simulink model "YMC_vicrt"  (R2021a)
settings: Solver=ode4  StartTime=0.0  StopTime=inf  FixedStep=0.001  RelTol=1e-3
model workspace (MAT data in the model file):
  inChnlList : object (value not decoded)
  inChnlListInternal : object (value not decoded)
  outChnlList : object (value not decoded)
  outChnlListInternal : object (value not decoded)
values from neighbouring files (symbols this model uses):
  a = (1-wb)*w    (= 0.84425)    [YMC_launcherVICRT.m]
  b = w-a    (= 0.69075)    [YMC_launcherVICRT.m]
  BP = 1*2*pi    (= 6.28318530718)    [YMC_launcherVICRT.m]
  brakeVector = throttleVector    [YMC_launcherVICRT.m]    (also in motorMaps.m)
  Cf = 515.7027*180/pi    (= 29547.5881935)    [YMC_launcherVICRT.m]
  Cr = 630.3033*180/pi    (= 36113.7189032)    [YMC_launcherVICRT.m]
  g = 9.81    [YMC_launcherVICRT.m]
  Izz = 112.4    [YMC_launcherVICRT.m]
  m = 272    [YMC_launcherVICRT.m]
  maxYMC = maxForceAtWheel *0.4 * (tFront + tRear)    (= 1272.43505906)    [YMC_launcherVICRT.m]
  nominalWheelRadius = 0.2032    [YMC_launcherVICRT.m]
  omegaLP = 2*pi*freqLP    (= 157.079632679)    [YMC_launcherVICRT.m]
  phaseMargin = deg2rad(90)    [YMC_launcherVICRT.m]
  speedVector = linspace(0,wmax,nPoints)    [YMC_launcherVICRT.m]    (also in motorMaps.m = linspace(0,mot.limit.wmax,nPoints))
  steerFront = [-95 -92.2857142857 -89.5714285714 -86.8571428571 -84.1428571429 -81.4285714286 -78.7142857143 -76 -73.2857142857 -70.5714285714 -67.8571428571 -65.1428571429 ... (213 elements, 71x3)]    [steerFront.mat]
  taregtKUS = 0.02    [YMC_launcherVICRT.m]
  tau = 12.667    [YMC_launcherVICRT.m]
  Tc = 1e-3    (= 0.001)    [YMC_launcherVICRT.m]
  tFront = 1.23    [YMC_launcherVICRT.m]
  TorqueFront = TorqueRear * vehicle.setup.frontTorqueFactor    [motorMaps.m]    (also in torqueMaps.mat = [0 0 0 0 0 0 0 0 0 0 0 0 ... (1071 elements, 51x21)])
  TorqueFrontRegen = zeros(nPoints,nPointsPedals)    [motorMaps.m]    (also in torqueMaps.mat = [0 0 0 0 0 0 0 0 0 0 0 0 ... (1071 elements, 51x21)])
  TorqueLimit = zeros(nPoints,1)    [motorMaps.m]    (also in torqueMaps.mat = [21 21 21 21 21 21 21 21 21 21 21 21 ... (51 elements, 51x1))
  TorqueRear = zeros(nPoints,nPointsPedals)    [motorMaps.m]    (also in torqueMaps.mat = [0 0 0 0 0 0 0 0 0 0 0 0 ... (1071 elements, 51x21)])
  TorqueRearRegen = TorqueFrontRegen * vehicle.setup.rearRegenFactor    [motorMaps.m]    (also in torqueMaps.mat = [0 0 0 0 0 0 0 0 0 0 0 0 ... (1071 elements, 51x21)])
  tRear = 1.2    [YMC_launcherVICRT.m]
  w = 1.535    [YMC_launcherVICRT.m]
undefined symbols (not defined in the file or in its folder): ki, kp
libraries: simwbSfunlib x42, slpidlib x1
settings Model: Creator=Alber  LastModifiedBy=User
settings DataIOCC: ReturnWorkspaceOutputsName=outVICRT
settings DebuggingCC: UnconnectedInputMsg=none  UnconnectedOutputMsg=none  UnconnectedLineMsg=none
settings ModelReferenceCC: EnableRefExpFcnMdlSchedulingChecks=off
settings RTWCC: Description=VI-CarRealTime Solver Plugin V1.0  SystemTargetFile=vicrt_plugin.tlc  TemplateMakefile=vicrt_plugin_mingw64.tmf  PostCodeGenCommand=if strcmp(get_param(bdroot,'TemplateMakefile'),'vicrt_plugin_ccur.tmf'),copyfile([matlabroot,filesep,'rtw',filesep,'c',filesep,'tools',filesep,'unixtools.mk'],'unixtools.mk'),if ~verLessThan('matlab','9.6'),set_param(bdroot,'MatFileLogging','off'),end,end  DLArmComputeVersion=20.02.1
settings CodeAppCC: MaxIdLength=80
settings STFCustomTargetCC: TargetLangStandard=C99 (ISO)  ModelReferenceCompliant=off  CombineOutputUpdateFcns=on  MatFileLogging=on  GRTInterface=off  UseToolchainInfoCompliant=off  SystemTargetFile=vicrt_plugin.tlc
settings GRTTargetCC: ModelReferenceCompliant=off  ParMdlRefBuildCompliant=off  CompOptLevelCompliant=off  ConcurrentExecutionCompliant=off  CPPClassGenCompliant=off  UseToolchainInfoCompliant=off  RTWCAPIParams=on

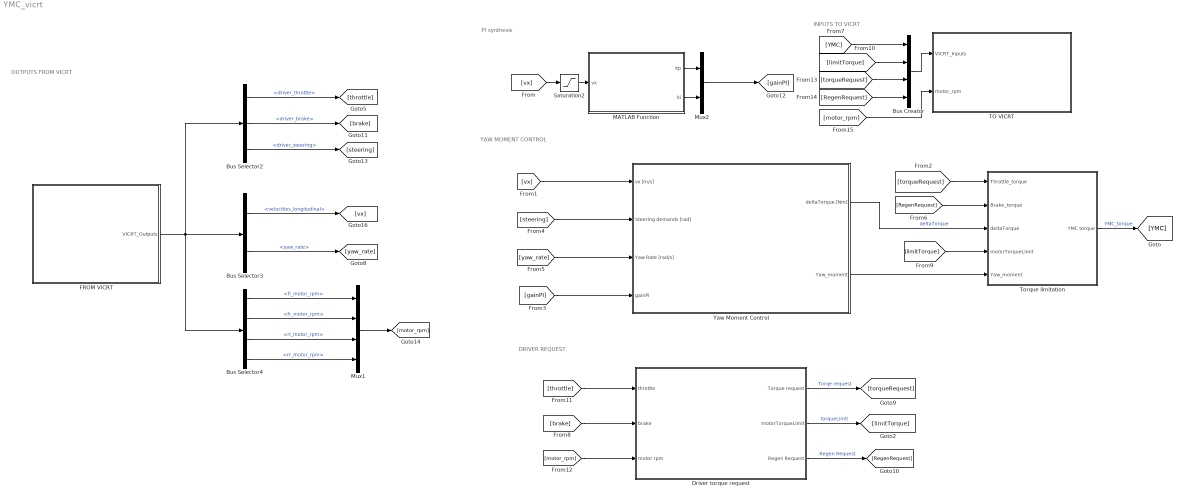
== system YMC_vicrt ==
  note: INPUTS TO VICRT
  note: OUTPUTS FROM VICRT
  note: PI synthesis
  note: DRIVER REQUEST
  note: YAW MOMENT CONTROL
  Bus Creator : BusCreator  Inputs=4
  Bus Selector2 : BusSelector  OutputSignals=driver_throttle,driver_brake,driver_steering
  Bus Selector3 : BusSelector  OutputSignals=velocities_longitudinal,yaw_rate
  Bus Selector4 : BusSelector  OutputSignals=fl_motor_rpm,fr_motor_rpm,rl_motor_rpm,rr_motor_rpm
  Driver torque request : Subsystem
  FROM VICRT : Subsystem
  MATLAB Function : MATLAB Function  TreatAsAtomicUnit=on
  Mux1 : Mux
  Mux2 : Mux  Inputs=2
  Saturation2 : Saturate  UpperLimit=inf  LowerLimit=1
  TO VICRT : Subsystem
  Torque limitation : Subsystem
  Yaw Moment Control : Subsystem
  wires:
  Driver torque request/2(motorTorqueLimit) -> [limitTorque]  "torqueLimit"
  MATLAB Function/2(ki) -> Mux2/2
  MATLAB Function/1(kp) -> Mux2/1
  Yaw Moment Control/1(deltaTorque [Nm]) -> Torque limitation/3(deltaTorque)  "deltaTorque"
  Torque limitation/1(YMC torque) -> [YMC]  "YMC_torque"
  [limitTorque] -> Torque limitation/4(motorTorqueLimit)
  Driver torque request/1(Torque request) -> [torqueRequest]  "Torqe request"
  Mux2/1 -> [gainPI]
  [vx] -> Saturation2/1
  Saturation2/1 -> MATLAB Function/1(vx)
  [gainPI] -> Yaw Moment Control/4("gainPI ")
  Bus Selector2/1 -> [throttle]  "<driver_throttle>"
  Bus Selector2/2 -> [brake]  "<driver_brake>"
  Bus Selector2/3 -> [steering]  "<driver_steering>"
  Bus Selector3/1 -> [vx]  "<velocities_longitudinal>"
  Bus Selector3/2 -> [yaw_rate]  "<yaw_rate>"
  FROM VICRT/1(VICRT_Outputs) -> Bus Selector4/1, Bus Selector3/1, Bus Selector2/1
  Bus Selector4/3 -> Mux1/3  "<rl_motor_rpm>"
  Bus Selector4/1 -> Mux1/1  "<fl_motor_rpm>"
  Bus Selector4/2 -> Mux1/2  "<fr_motor_rpm>"
  Bus Selector4/4 -> Mux1/4  "<rr_motor_rpm>"
  Mux1/1 -> [motor_rpm]
  [vx] -> Yaw Moment Control/1(vx [m/s])
  [yaw_rate] -> Yaw Moment Control/3(Yaw Rate [rad/s])
  [steering] -> Yaw Moment Control/2(Steering demands [rad])
  Driver torque request/3(Regen Request) -> [RegenRequest]  "Regen Request"
  [brake] -> Driver torque request/2(brake)
  [throttle] -> Driver torque request/1(throttle)
  [motor_rpm] -> Driver torque request/3(motor rpm)
  [torqueRequest] -> Torque limitation/1(Throttle_torque)
  [RegenRequest] -> Torque limitation/2(Brake_torque)
  [YMC] -> Bus Creator/1
  Bus Creator/1 -> TO VICRT/1(VICRT_Inputs)
  [limitTorque] -> Bus Creator/2
  Yaw Moment Control/2(Yaw_moment) -> Torque limitation/5(Yaw_moment)
  [torqueRequest] -> Bus Creator/3
  [RegenRequest] -> Bus Creator/4
  [motor_rpm] -> TO VICRT/2(motor_rpm)

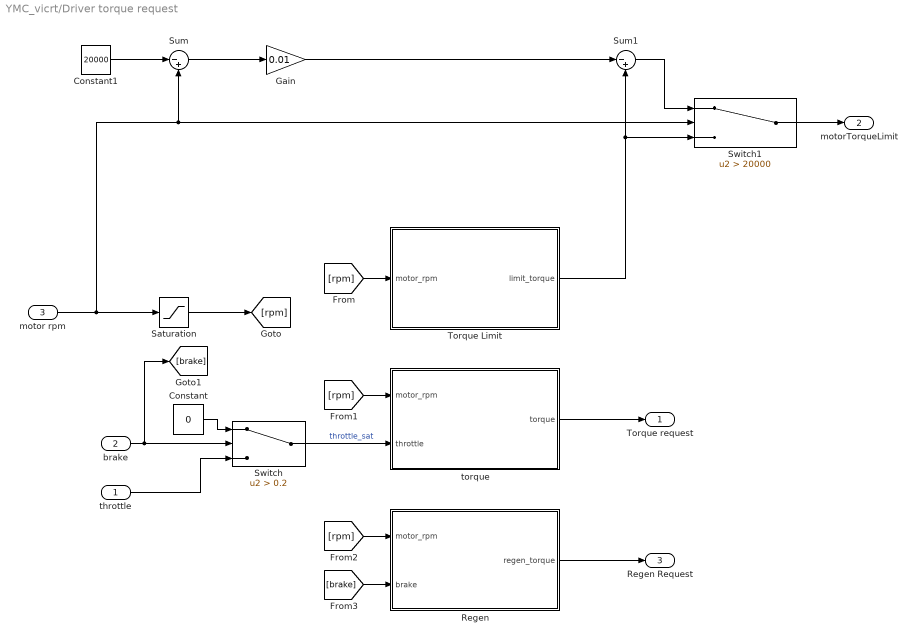
== system YMC_vicrt/Driver torque request ==
  throttle : Inport
  brake : Inport  Port=2
  motor rpm : Inport  Port=3
  Constant : Constant  Value=0
  Constant1 : Constant  Value=20000
  Gain : Gain  Gain=0.01
  Regen : Subsystem
  Saturation : Saturate  UpperLimit=20000  LowerLimit=0
  Sum : Sum  Inputs=|-+
  Sum1 : Sum  Inputs=|-+
  Switch : Switch  Criteria=u2 > Threshold  Threshold=0.2
  Switch1 : Switch  Criteria=u2 > Threshold  Threshold=20000
  Torque Limit : Subsystem
  torque : Subsystem
  Torque request : Outport
  motorTorqueLimit : Outport  Port=2
  Regen Request : Outport  Port=3
  wires:
  motor rpm/1 -> Sum/2, Switch1/2, Saturation/1
  [rpm] -> Torque Limit/1(motor_rpm)
  [rpm] -> torque/1(motor_rpm)
  [rpm] -> Regen/1(motor_rpm)
  Regen/1(regen_torque) -> Regen Request/1
  torque/1(torque) -> Torque request/1
  brake/1 -> Switch/2, [brake]
  Switch/1 -> torque/2(throttle)  "throttle_sat"
  [brake] -> Regen/2(brake)
  throttle/1 -> Switch/3
  Constant/1 -> Switch/1
  Saturation/1 -> [rpm]
  Constant1/1 -> Sum/1
  Sum/1 -> Gain/1
  Gain/1 -> Sum1/1
  Sum1/1 -> Switch1/1
  Switch1/1 -> motorTorqueLimit/1
  Torque Limit/1(limit_torque) -> Switch1/3, Sum1/2

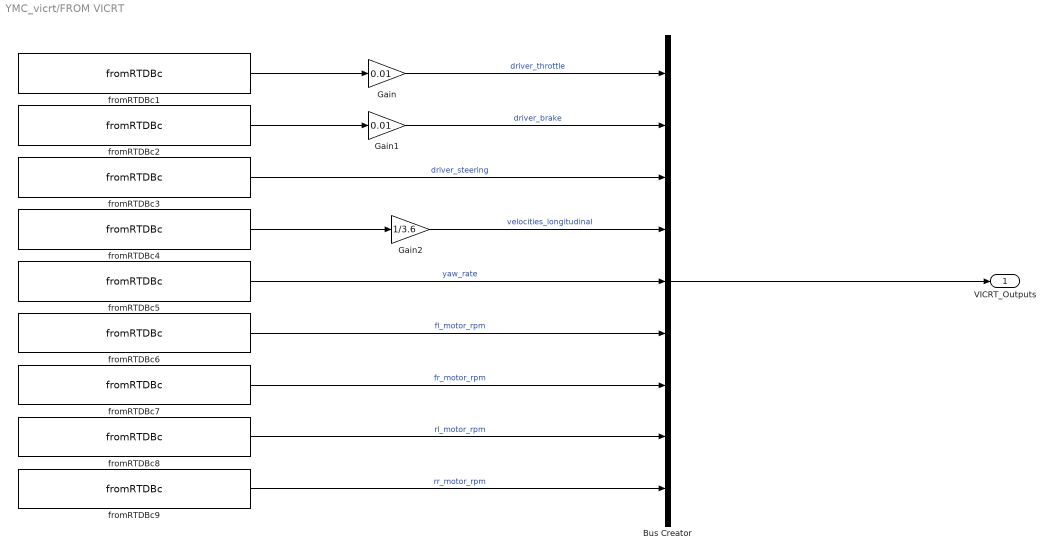
== system YMC_vicrt/FROM VICRT ==
  Bus Creator : BusCreator  Inputs=9
  Gain : Gain  Gain=0.01
  Gain1 : Gain  Gain=0.01
  Gain2 : Gain  Gain=1/3.6
  fromRTDBc1 : simwbSfunlib/fromRTDBc  stringBlock=off  varName=VI_CarRealTime.Outputs.driver_demands.throttle  sigDim=[1 1]  sigType=double  sampleTime=[-1 0]  maxBuffSize=1024  busName=nobus  defaultValue=0  defaultString=simwbin  hasMapping=0  ptrName=VI_CarRealTime_Outputs_driver_demands_throttle  enumOrAlias=nothing
      settings: SourceProductName=SimWB MLToolkit
  fromRTDBc2 : simwbSfunlib/fromRTDBc  stringBlock=off  varName=VI_CarRealTime.Outputs.driver_demands.brake  sigDim=[1 1]  sigType=double  sampleTime=[-1 0]  maxBuffSize=1024  busName=nobus  defaultValue=0  defaultString=simwbin  hasMapping=0  ptrName=VI_CarRealTime_Outputs_driver_demands_brake  enumOrAlias=nothing
      settings: SourceProductName=SimWB MLToolkit
  fromRTDBc3 : simwbSfunlib/fromRTDBc  stringBlock=off  varName=VI_CarRealTime.Outputs.driver_demands.steering  sigDim=[1 1]  sigType=double  sampleTime=[-1 0]  maxBuffSize=1024  busName=nobus  defaultValue=0  defaultString=simwbin  hasMapping=0  ptrName=VI_CarRealTime_Outputs_driver_demands_steering  enumOrAlias=nothing
      settings: SourceProductName=SimWB MLToolkit
  fromRTDBc4 : simwbSfunlib/fromRTDBc  stringBlock=off  varName=VI_CarRealTime.Outputs.chassis_velocities.longitudinal  sigDim=[1 1]  sigType=double  sampleTime=[-1 0]  maxBuffSize=1024  busName=nobus  defaultValue=0  defaultString=simwbin  hasMapping=0  ptrName=VI_CarRealTime_Outputs_chassis_velocities_longitudinal  enumOrAlias=nothing
      settings: SourceProductName=SimWB MLToolkit
  fromRTDBc5 : simwbSfunlib/fromRTDBc  stringBlock=off  varName=VI_CarRealTime.Outputs.chassis_velocities.yaw  sigDim=[1 1]  sigType=double  sampleTime=[-1 0]  maxBuffSize=1024  busName=nobus  defaultValue=0  defaultString=simwbin  hasMapping=0  ptrName=VI_CarRealTime_Outputs_chassis_velocities_yaw  enumOrAlias=nothing
      settings: SourceProductName=SimWB MLToolkit
  fromRTDBc6 : simwbSfunlib/fromRTDBc  stringBlock=off  varName=VI_CarRealTime.Outputs.motor_to_front_left_wheel.engine_rpm  sigDim=[1 1]  sigType=double  sampleTime=[-1 0]  maxBuffSize=1024  busName=nobus  defaultValue=0  defaultString=simwbin  hasMapping=0  ptrName=VI_CarRealTime_Outputs_motor_to_front_left_wheel_engine_rpm  enumOrAlias=nothing
      settings: SourceProductName=SimWB MLToolkit
  fromRTDBc7 : simwbSfunlib/fromRTDBc  stringBlock=off  varName=VI_CarRealTime.Outputs.motor_to_front_right_wheel.engine_rpm  sigDim=[1 1]  sigType=double  sampleTime=[-1 0]  maxBuffSize=1024  busName=nobus  defaultValue=0  defaultString=simwbin  hasMapping=0  ptrName=VI_CarRealTime_Outputs_motor_to_front_right_wheel_engine_rpm  enumOrAlias=nothing
      settings: SourceProductName=SimWB MLToolkit
  fromRTDBc8 : simwbSfunlib/fromRTDBc  stringBlock=off  varName=VI_CarRealTime.Outputs.motor_to_rear_left_wheel.engine_rpm  sigDim=[1 1]  sigType=double  sampleTime=[-1 0]  maxBuffSize=1024  busName=nobus  defaultValue=0  defaultString=simwbin  hasMapping=0  ptrName=VI_CarRealTime_Outputs_motor_to_rear_left_wheel_engine_rpm  enumOrAlias=nothing
      settings: SourceProductName=SimWB MLToolkit
  fromRTDBc9 : simwbSfunlib/fromRTDBc  stringBlock=off  varName=VI_CarRealTime.Outputs.motor_to_rear_right_wheel.engine_rpm  sigDim=[1 1]  sigType=double  sampleTime=[-1 0]  maxBuffSize=1024  busName=nobus  defaultValue=0  defaultString=simwbin  hasMapping=0  ptrName=VI_CarRealTime_Outputs_motor_to_rear_right_wheel_engine_rpm  enumOrAlias=nothing
      settings: SourceProductName=SimWB MLToolkit
  VICRT_Outputs : Outport
  wires:
  Bus Creator/1 -> VICRT_Outputs/1
  fromRTDBc1/1 -> Gain/1
  Gain/1 -> Bus Creator/1  "driver_throttle"
  fromRTDBc2/1 -> Gain1/1
  Gain1/1 -> Bus Creator/2  "driver_brake"
  fromRTDBc3/1 -> Bus Creator/3  "driver_steering"
  fromRTDBc5/1 -> Bus Creator/5  "yaw_rate"
  fromRTDBc4/1 -> Gain2/1
  Gain2/1 -> Bus Creator/4  "velocities_longitudinal"
  fromRTDBc6/1 -> Bus Creator/6  "fl_motor_rpm"
  fromRTDBc7/1 -> Bus Creator/7  "fr_motor_rpm"
  fromRTDBc8/1 -> Bus Creator/8  "rl_motor_rpm"
  fromRTDBc9/1 -> Bus Creator/9  "rr_motor_rpm"

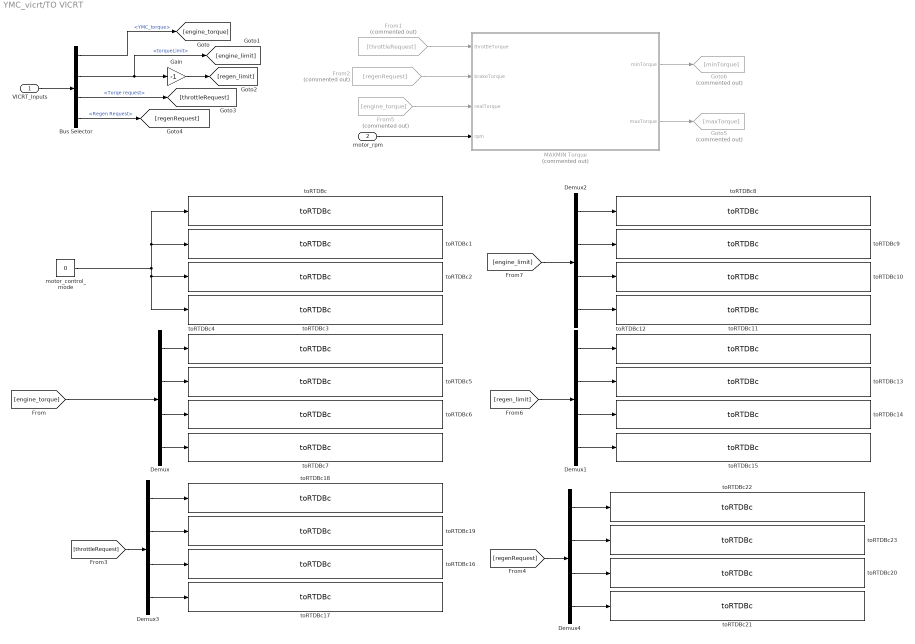
== system YMC_vicrt/TO VICRT ==
  VICRT_Inputs : Inport
  motor_rpm : Inport  Port=2
  Bus Selector : BusSelector  OutputSignals=YMC_torque,torqueLimit,Torqe request,Regen Request
  Demux{,1..4} (5 alike) : Demux
  From1 : From  Commented=on  GotoTag=throttleRequest
  From2 : From  Commented=on  GotoTag=regenRequest
  From5 : From  Commented=on  GotoTag=engine_torque
  Gain : Gain  Gain=-1
  Goto5 : Goto  Commented=on  GotoTag=maxTorque
  Goto6 : Goto  Commented=on  GotoTag=minTorque
  MAXMIN Torque : Subsystem  Commented=on
  motor_control_mode : Constant  Value=0
  toRTDBc : simwbSfunlib/toRTDBc  stringBlock=off  varName=VI_CarRealTime.Inputs.Subsystem_Activation.Internal_Motor_to_FrontLeftWheel_Activity  sigDim=[1 1]  sigType=double  sampleTime=[-1 0]  maxBuffSize=1024  busName=nobus  defaultValue=0  defaultString=simwbout  hasMapping=0  ptrName=VI_CarRealTime_Inputs_Subsystem_Activation_Internal_Motor_to_FrontLeftWheel_Activity  enumOrAlias=nothing
      settings: SourceProductName=SimWB MLToolkit
  toRTDBc1 : simwbSfunlib/toRTDBc  stringBlock=off  varName=VI_CarRealTime.Inputs.Subsystem_Activation.Internal_Motor_to_FrontRightWheel_Activity  sigDim=[1 1]  sigType=double  sampleTime=[-1 0]  maxBuffSize=1024  busName=nobus  defaultValue=0  defaultString=simwbout  hasMapping=0  ptrName=VI_CarRealTime_Inputs_Subsystem_Activation_Internal_Motor_to_FrontRightWheel_Activity  enumOrAlias=nothing
      settings: SourceProductName=SimWB MLToolkit
  toRTDBc10 : simwbSfunlib/toRTDBc  stringBlock=off  varName=VI_CarRealTime.Inputs.Generic_Engine_to_Rear_Left_Wheel.engine_max_torque  sigDim=[1 1]  sigType=double  sampleTime=[-1 0]  maxBuffSize=1024  busName=nobus  defaultValue=0  defaultString=simwbout  hasMapping=0  ptrName=VI_CarRealTime_Inputs_Generic_Engine_to_Rear_Left_Wheel_engine_max_torque  enumOrAlias=nothing
      settings: SourceProductName=SimWB MLToolkit
  toRTDBc11 : simwbSfunlib/toRTDBc  stringBlock=off  varName=VI_CarRealTime.Inputs.Generic_Engine_to_Rear_Right_Wheel.engine_max_torque  sigDim=[1 1]  sigType=double  sampleTime=[-1 0]  maxBuffSize=1024  busName=nobus  defaultValue=0  defaultString=simwbout  hasMapping=0  ptrName=VI_CarRealTime_Inputs_Generic_Engine_to_Rear_Right_Wheel_engine_max_torque  enumOrAlias=nothing
      settings: SourceProductName=SimWB MLToolkit
  toRTDBc12 : simwbSfunlib/toRTDBc  stringBlock=off  varName=VI_CarRealTime.Inputs.Generic_Engine_to_Front_Left_Wheel.engine_min_torque  sigDim=[1 1]  sigType=double  sampleTime=[-1 0]  maxBuffSize=1024  busName=nobus  defaultValue=0  defaultString=simwbout  hasMapping=0  ptrName=VI_CarRealTime_Inputs_Generic_Engine_to_Front_Left_Wheel_engine_min_torque  enumOrAlias=nothing
      settings: SourceProductName=SimWB MLToolkit
  toRTDBc13 : simwbSfunlib/toRTDBc  stringBlock=off  varName=VI_CarRealTime.Inputs.Generic_Engine_to_Front_Right_Wheel.engine_min_torque  sigDim=[1 1]  sigType=double  sampleTime=[-1 0]  maxBuffSize=1024  busName=nobus  defaultValue=0  defaultString=simwbout  hasMapping=0  ptrName=VI_CarRealTime_Inputs_Generic_Engine_to_Front_Right_Wheel_engine_min_torque  enumOrAlias=nothing
      settings: SourceProductName=SimWB MLToolkit
  toRTDBc14 : simwbSfunlib/toRTDBc  stringBlock=off  varName=VI_CarRealTime.Inputs.Generic_Engine_to_Rear_Left_Wheel.engine_min_torque  sigDim=[1 1]  sigType=double  sampleTime=[-1 0]  maxBuffSize=1024  busName=nobus  defaultValue=0  defaultString=simwbout  hasMapping=0  ptrName=VI_CarRealTime_Inputs_Generic_Engine_to_Rear_Left_Wheel_engine_min_torque  enumOrAlias=nothing
      settings: SourceProductName=SimWB MLToolkit
  toRTDBc15 : simwbSfunlib/toRTDBc  stringBlock=off  varName=VI_CarRealTime.Inputs.Generic_Engine_to_Rear_Right_Wheel.engine_min_torque  sigDim=[1 1]  sigType=double  sampleTime=[-1 0]  maxBuffSize=1024  busName=nobus  defaultValue=0  defaultString=simwbout  hasMapping=0  ptrName=VI_CarRealTime_Inputs_Generic_Engine_to_Rear_Right_Wheel_engine_min_torque  enumOrAlias=nothing
      settings: SourceProductName=SimWB MLToolkit
  toRTDBc16 : simwbSfunlib/toRTDBc  stringBlock=off  varName=YMC.torqueRequest.RL  sigDim=[1 1]  sigType=double  sampleTime=[-1 0]  maxBuffSize=1024  busName=nobus  defaultValue=0  defaultString=simwbout  hasMapping=0  ptrName=YMC_torqueRequest_RL  enumOrAlias=nothing
      settings: SourceProductName=SimWB MLToolkit
  toRTDBc17 : simwbSfunlib/toRTDBc  stringBlock=off  varName=YMC.torqueRequest.RR  sigDim=[1 1]  sigType=double  sampleTime=[-1 0]  maxBuffSize=1024  busName=nobus  defaultValue=0  defaultString=simwbout  hasMapping=0  ptrName=YMC_torqueRequest_RR  enumOrAlias=nothing
      settings: SourceProductName=SimWB MLToolkit
  toRTDBc18 : simwbSfunlib/toRTDBc  stringBlock=off  varName=YMC.torqueRequest.FL  sigDim=[1 1]  sigType=double  sampleTime=[-1 0]  maxBuffSize=1024  busName=nobus  defaultValue=0  defaultString=simwbout  hasMapping=0  ptrName=YMC_torqueRequest_FL  enumOrAlias=nothing
      settings: SourceProductName=SimWB MLToolkit
  toRTDBc19 : simwbSfunlib/toRTDBc  stringBlock=off  varName=YMC.torqueRequest.FR  sigDim=[1 1]  sigType=double  sampleTime=[-1 0]  maxBuffSize=1024  busName=nobus  defaultValue=0  defaultString=simwbout  hasMapping=0  ptrName=YMC_torqueRequest_FR  enumOrAlias=nothing
      settings: SourceProductName=SimWB MLToolkit
  toRTDBc2 : simwbSfunlib/toRTDBc  stringBlock=off  varName=VI_CarRealTime.Inputs.Subsystem_Activation.Internal_Motor_to_RearLeftWheel_Activity  sigDim=[1 1]  sigType=double  sampleTime=[-1 0]  maxBuffSize=1024  busName=nobus  defaultValue=0  defaultString=simwbout  hasMapping=0  ptrName=VI_CarRealTime_Inputs_Subsystem_Activation_Internal_Motor_to_RearLeftWheel_Activity  enumOrAlias=nothing
      settings: SourceProductName=SimWB MLToolkit
  toRTDBc20 : simwbSfunlib/toRTDBc  stringBlock=off  varName=YMC.regenRequest.RL  sigDim=[1 1]  sigType=double  sampleTime=[-1 0]  maxBuffSize=1024  busName=nobus  defaultValue=0  defaultString=simwbout  hasMapping=0  ptrName=YMC_regenRequest_RL  enumOrAlias=nothing
      settings: SourceProductName=SimWB MLToolkit
  toRTDBc21 : simwbSfunlib/toRTDBc  stringBlock=off  varName=YMC.regenRequest.RR  sigDim=[1 1]  sigType=double  sampleTime=[-1 0]  maxBuffSize=1024  busName=nobus  defaultValue=0  defaultString=simwbout  hasMapping=0  ptrName=YMC_regenRequest_RR  enumOrAlias=nothing
      settings: SourceProductName=SimWB MLToolkit
  toRTDBc22 : simwbSfunlib/toRTDBc  stringBlock=off  varName=YMC.regenRequest.FL  sigDim=[1 1]  sigType=double  sampleTime=[-1 0]  maxBuffSize=1024  busName=nobus  defaultValue=0  defaultString=simwbout  hasMapping=0  ptrName=YMC_regenRequest_FL  enumOrAlias=nothing
      settings: SourceProductName=SimWB MLToolkit
  toRTDBc23 : simwbSfunlib/toRTDBc  stringBlock=off  varName=YMC.regenRequest.FR  sigDim=[1 1]  sigType=double  sampleTime=[-1 0]  maxBuffSize=1024  busName=nobus  defaultValue=0  defaultString=simwbout  hasMapping=0  ptrName=YMC_regenRequest_FR  enumOrAlias=nothing
      settings: SourceProductName=SimWB MLToolkit
  toRTDBc3 : simwbSfunlib/toRTDBc  stringBlock=off  varName=VI_CarRealTime.Inputs.Subsystem_Activation.Internal_Motor_to_RearRightWheel_Activity  sigDim=[1 1]  sigType=double  sampleTime=[-1 0]  maxBuffSize=1024  busName=nobus  defaultValue=0  defaultString=simwbout  hasMapping=0  ptrName=VI_CarRealTime_Inputs_Subsystem_Activation_Internal_Motor_to_RearRightWheel_Activity  enumOrAlias=nothing
      settings: SourceProductName=SimWB MLToolkit
  toRTDBc4 : simwbSfunlib/toRTDBc  stringBlock=off  varName=VI_CarRealTime.Inputs.Generic_Engine_to_Front_Left_Wheel.engine_torque  sigDim=[1 1]  sigType=double  sampleTime=[-1 0]  maxBuffSize=1024  busName=nobus  defaultValue=0  defaultString=simwbout  hasMapping=0  ptrName=VI_CarRealTime_Inputs_Generic_Engine_to_Front_Left_Wheel_engine_torque  enumOrAlias=nothing
      settings: SourceProductName=SimWB MLToolkit
  toRTDBc5 : simwbSfunlib/toRTDBc  stringBlock=off  varName=VI_CarRealTime.Inputs.Generic_Engine_to_Front_Right_Wheel.engine_torque  sigDim=[1 1]  sigType=double  sampleTime=[-1 0]  maxBuffSize=1024  busName=nobus  defaultValue=0  defaultString=simwbout  hasMapping=0  ptrName=VI_CarRealTime_Inputs_Generic_Engine_to_Front_Right_Wheel_engine_torque  enumOrAlias=nothing
      settings: SourceProductName=SimWB MLToolkit
  toRTDBc6 : simwbSfunlib/toRTDBc  stringBlock=off  varName=VI_CarRealTime.Inputs.Generic_Engine_to_Rear_Left_Wheel.engine_torque  sigDim=[1 1]  sigType=double  sampleTime=[-1 0]  maxBuffSize=1024  busName=nobus  defaultValue=0  defaultString=simwbout  hasMapping=0  ptrName=VI_CarRealTime_Inputs_Generic_Engine_to_Rear_Left_Wheel_engine_torque  enumOrAlias=nothing
      settings: SourceProductName=SimWB MLToolkit
  toRTDBc7 : simwbSfunlib/toRTDBc  stringBlock=off  varName=VI_CarRealTime.Inputs.Generic_Engine_to_Rear_Right_Wheel.engine_torque  sigDim=[1 1]  sigType=double  sampleTime=[-1 0]  maxBuffSize=1024  busName=nobus  defaultValue=0  defaultString=simwbout  hasMapping=0  ptrName=VI_CarRealTime_Inputs_Generic_Engine_to_Rear_Right_Wheel_engine_torque  enumOrAlias=nothing
      settings: SourceProductName=SimWB MLToolkit
  toRTDBc8 : simwbSfunlib/toRTDBc  stringBlock=off  varName=VI_CarRealTime.Inputs.Generic_Engine_to_Front_Left_Wheel.engine_max_torque  sigDim=[1 1]  sigType=double  sampleTime=[-1 0]  maxBuffSize=1024  busName=nobus  defaultValue=0  defaultString=simwbout  hasMapping=0  ptrName=VI_CarRealTime_Inputs_Generic_Engine_to_Front_Left_Wheel_engine_max_torque  enumOrAlias=nothing
      settings: SourceProductName=SimWB MLToolkit
  toRTDBc9 : simwbSfunlib/toRTDBc  stringBlock=off  varName=VI_CarRealTime.Inputs.Generic_Engine_to_Front_Right_Wheel.engine_max_torque  sigDim=[1 1]  sigType=double  sampleTime=[-1 0]  maxBuffSize=1024  busName=nobus  defaultValue=0  defaultString=simwbout  hasMapping=0  ptrName=VI_CarRealTime_Inputs_Generic_Engine_to_Front_Right_Wheel_engine_max_torque  enumOrAlias=nothing
      settings: SourceProductName=SimWB MLToolkit
  wires:
  VICRT_Inputs/1 -> Bus Selector/1
  motor_control_mode/1 -> toRTDBc1/1, toRTDBc/1, toRTDBc3/1, toRTDBc2/1
  Bus Selector/1 -> [engine_torque]  "<YMC_torque>"
  Bus Selector/2 -> [engine_limit], Gain/1  "<torqueLimit>"
  Demux/1 -> toRTDBc4/1
  Demux/2 -> toRTDBc5/1
  Demux/3 -> toRTDBc6/1
  Demux/4 -> toRTDBc7/1
  Demux1/4 -> toRTDBc15/1
  Demux1/2 -> toRTDBc13/1
  Demux1/3 -> toRTDBc14/1
  Demux1/1 -> toRTDBc12/1
  Demux2/4 -> toRTDBc11/1
  Demux2/3 -> toRTDBc10/1
  Demux2/2 -> toRTDBc9/1
  Demux2/1 -> toRTDBc8/1
  Gain/1 -> [regen_limit]
  [regen_limit] -> Demux1/1
  [engine_limit] -> Demux2/1
  Bus Selector/3 -> [throttleRequest]  "<Torqe request>"
  Bus Selector/4 -> [regenRequest]  "<Regen Request>"
  Demux3/2 -> toRTDBc19/1
  Demux3/4 -> toRTDBc17/1
  [throttleRequest] -> Demux3/1
  Demux3/3 -> toRTDBc16/1
  Demux3/1 -> toRTDBc18/1
  Demux4/2 -> toRTDBc23/1
  Demux4/1 -> toRTDBc22/1
  Demux4/3 -> toRTDBc20/1
  [regenRequest] -> Demux4/1
  Demux4/4 -> toRTDBc21/1
  From1/1 -> MAXMIN Torque/1(throttleTorque)
  From2/1 -> MAXMIN Torque/2(brakeTorque)
  From5/1 -> MAXMIN Torque/3(realTorque)
  motor_rpm/1 -> MAXMIN Torque/4(rpm)
  MAXMIN Torque/1(minTorque) -> Goto6/1
  MAXMIN Torque/2(maxTorque) -> Goto5/1
  [engine_torque] -> Demux/1

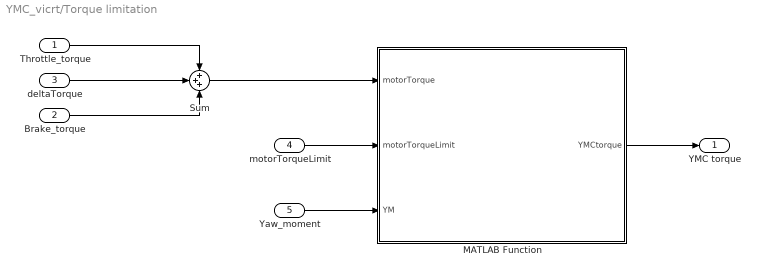
== system YMC_vicrt/Torque limitation ==
  Throttle_torque : Inport
  Brake_torque : Inport  Port=2
  deltaTorque : Inport  Port=3
  motorTorqueLimit : Inport  Port=4
  Yaw_moment : Inport  Port=5
  MATLAB Function : MATLAB Function  TreatAsAtomicUnit=on
  Sum : Sum  Inputs=+++
  YMC torque : Outport
  wires:
  motorTorqueLimit/1 -> MATLAB Function/2(motorTorqueLimit)
  Brake_torque/1 -> Sum/3
  deltaTorque/1 -> Sum/2
  Throttle_torque/1 -> Sum/1
  Sum/1 -> MATLAB Function/1(motorTorque)
  Yaw_moment/1 -> MATLAB Function/3(YM)
  MATLAB Function/1(YMCtorque) -> YMC torque/1

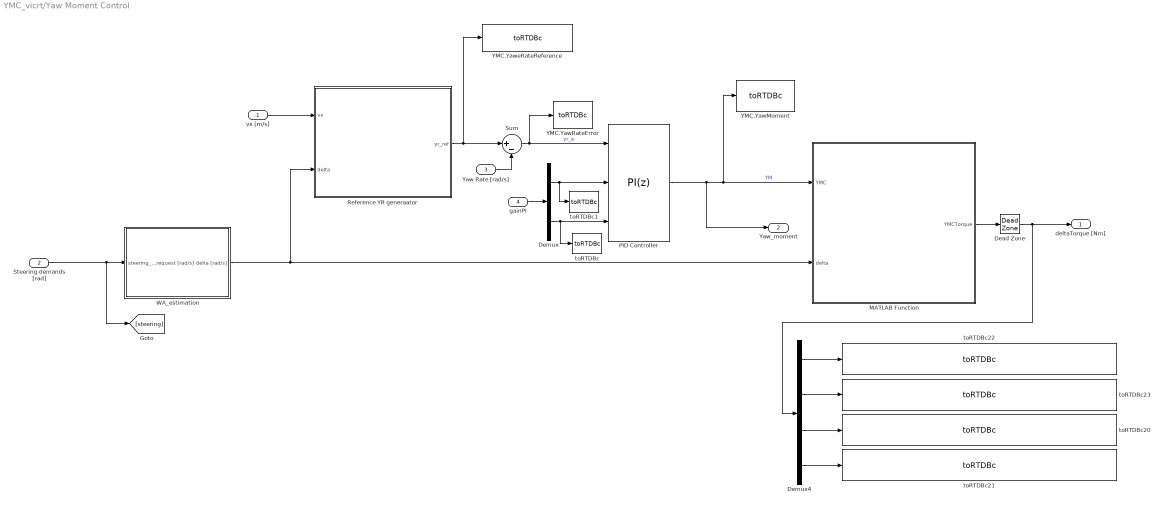
== system YMC_vicrt/Yaw Moment Control ==
  vx [m/s] : Inport
  Steering demands [rad] : Inport  Port=2
  Yaw Rate [rad/s] : Inport  Port=3
  "gainPI " : Inport  Port=4
  Dead Zone : DeadZone  LowerValue=-0.1  UpperValue=0.1  SaturateOnIntegerOverflow=on
  Demux : Demux  Outputs=2
  Demux4 : Demux
  MATLAB Function : MATLAB Function  TreatAsAtomicUnit=on
  PID Controller : slpidlib/PID Controller  Controller=PI  Form=Parallel  TimeDomain=Discrete-time  UseExternalTs=off  SampleTime=Tc  IntegratorMethod=Forward Euler  FilterMethod=Forward Euler  ControllerParametersSource=external  P=kp  I=ki  D=1  UseFilter=on  N=140.723674968444  TunerSelectOption=Transfer Function Based (PID Tuner App)  InitialConditionSource=internal  InitialConditionForIntegrator=0  InitialConditionForFilter=0  DifferentiatorICPrevScaledInput=0  ExternalReset=none  TrackingMode=off  Kt=1  LimitOutput=on  SatLimitsSource=internal  UpperSaturationLimit=1*maxYMC  LowerSaturationLimit=-1*maxYMC  LinearizeAsGain=off  AntiWindupMode=clamping  Kb=1  POutMin=[]  POutMax=[]  IOutMin=[]  IOutMax=[]  DOutMin=[]  DOutMax=[]  NOutMin=[]  NOutMax=[]  SumOutMin=[]  SumOutMax=[]  SaturationOutMin=[]  SaturationOutMax=[]  PParamMin=[]  PParamMax=[]  IParamMin=[]  IParamMax=[]  DParamMin=[]  DParamMax=[]  NParamMin=[]  NParamMax=[]  KbParamMin=[]  KbParamMax=[]  KtParamMin=[]  KtParamMax=[]  KbOutMin=[]  KbOutMax=[]  KtOutMin=[]  KtOutMax=[]  IntegratorOutMin=[]  IntegratorOutMax=[]  FilterOutMin=[]  FilterOutMax=[]  SumI1OutMin=[]  SumI1OutMax=[]  SumI2OutMin=[]  SumI2OutMax=[]  SumI3OutMin=[]  SumI3OutMax=[]  SumI4OutMin=[]  SumI4OutMax=[]  SumDOutMin=[]  SumDOutMax=[]  DifferentiatorOutMin=[]  DifferentiatorOutMax=[]  FilterDiffOutCoefMin=[]  FilterDiffOutCoefMax=[]  ReciprocalOutMin=[]  ReciprocalOutMax=[]  SumDenOutMin=[]  SumDenOutMax=[]  SumNumOutMin=[]  SumNumOutMax=[]  DivideOutMin=[]  DivideOutMax=[]  UdiffTsProdOutMin=[]  UdiffTsProdOutMax=[]  NTsProdOutMin=[]  NTsProdOutMax=[]  UintegralTsProdOutMin=[]  UintegralTsProdOutMax=[]  UngainTsProdOutMin=[]  UngainTsProdOutMax=[]  IntegratorContinuousStateAttributes=''  IntegratorStateMustResolveToSignalObject=off  IntegratorRTWStateStorageClass=Auto  FilterContinuousStateAttributes=''  FilterStateMustResolveToSignalObject=off  FilterRTWStateStorageClass=Auto  ParallelPVariant=ExternalParameters  IdealPVariant=Disabled  IVariant=ExternalParameters  DVariant=Disabled  IntegratorVariant=Discrete  SatVariant=Enabled  AWVariant=DiscClampingParallel  PCopyVariant=Disabled  TRVariant=Disabled  FdbkBlocksVariant=Forward  IdealPFdbkVariant=Disabled  SatFdbkVariant=Disabled  DerivativeFilterVariant=Disabled  NVariant=Disabled  NCopyVariant=Disabled_SignalSpec  FilterICVariant=Disabled  IntegratorICVariant=InternalICs  ExternalResetVariant=Disabled  TRSumVariant=Passthrough  SumFdbkVariant=Disabled  SumVariant=Sum_PI  TsampFilterVariant=InternalTs  TsampNgainVariant=Passthrough  TsampIntegralVariant=Passthrough  ExternalSaturationOutDataTypeStr=Inherit: Same as second input
  Reference YR generaator : Subsystem
  Sum : Sum  Inputs=|+-
  WA_estimation : Subsystem
  YMC.YawMoment : simwbSfunlib/toRTDBc  stringBlock=off  varName=YMC.YawMoment  sigDim=[1 1]  sigType=double  sampleTime=[-1 0]  maxBuffSize=1024  busName=nobus  defaultValue=0  defaultString=simwbout  hasMapping=0  ptrName=YMC_YawMoment  enumOrAlias=nothing
      settings: SourceProductName=SimWB MLToolkit
  YMC.YawRateError : simwbSfunlib/toRTDBc  stringBlock=off  varName=YMC.YawRateError  sigDim=[1 1]  sigType=double  sampleTime=[-1 0]  maxBuffSize=1024  busName=nobus  defaultValue=0  defaultString=simwbout  hasMapping=0  ptrName=YMC_YawRateError  enumOrAlias=nothing
      settings: SourceProductName=SimWB MLToolkit
  YMC.YaweRateReference : simwbSfunlib/toRTDBc  stringBlock=off  varName=YMC.YawRateReference  sigDim=[1 1]  sigType=double  sampleTime=[-1 0]  maxBuffSize=1024  busName=nobus  defaultValue=0  defaultString=simwbout  hasMapping=0  ptrName=YMC_YawRateReference  enumOrAlias=nothing
      settings: SourceProductName=SimWB MLToolkit
  toRTDBc : simwbSfunlib/toRTDBc  stringBlock=off  varName=YMC.PI.ki  sigDim=[1 1]  sigType=double  sampleTime=[-1 0]  maxBuffSize=1024  busName=nobus  defaultValue=0  defaultString=simwbout  hasMapping=0  ptrName=YMC_PI_ki  enumOrAlias=nothing
      settings: SourceProductName=SimWB MLToolkit
  toRTDBc1 : simwbSfunlib/toRTDBc  stringBlock=off  varName=YMC.PI.kp  sigDim=[1 1]  sigType=double  sampleTime=[-1 0]  maxBuffSize=1024  busName=nobus  defaultValue=0  defaultString=simwbout  hasMapping=0  ptrName=YMC_PI_kp  enumOrAlias=nothing
      settings: SourceProductName=SimWB MLToolkit
  toRTDBc20 : simwbSfunlib/toRTDBc  stringBlock=off  varName=YMC.delta.RL  sigDim=[1 1]  sigType=double  sampleTime=[-1 0]  maxBuffSize=1024  busName=nobus  defaultValue=0  defaultString=simwbout  hasMapping=0  ptrName=YMC_delta_RL  enumOrAlias=nothing
      settings: SourceProductName=SimWB MLToolkit
  toRTDBc21 : simwbSfunlib/toRTDBc  stringBlock=off  varName=YMC.delta.RR  sigDim=[1 1]  sigType=double  sampleTime=[-1 0]  maxBuffSize=1024  busName=nobus  defaultValue=0  defaultString=simwbout  hasMapping=0  ptrName=YMC_delta_RR  enumOrAlias=nothing
      settings: SourceProductName=SimWB MLToolkit
  toRTDBc22 : simwbSfunlib/toRTDBc  stringBlock=off  varName=YMC.delta.FL  sigDim=[1 1]  sigType=double  sampleTime=[-1 0]  maxBuffSize=1024  busName=nobus  defaultValue=0  defaultString=simwbout  hasMapping=0  ptrName=YMC_delta_FL  enumOrAlias=nothing
      settings: SourceProductName=SimWB MLToolkit
  toRTDBc23 : simwbSfunlib/toRTDBc  stringBlock=off  varName=YMC.delta.FR  sigDim=[1 1]  sigType=double  sampleTime=[-1 0]  maxBuffSize=1024  busName=nobus  defaultValue=0  defaultString=simwbout  hasMapping=0  ptrName=YMC_delta_FR  enumOrAlias=nothing
      settings: SourceProductName=SimWB MLToolkit
  deltaTorque [Nm] : Outport
  Yaw_moment : Outport  Port=2
  wires:
  MATLAB Function/1(YMCTorque) -> Dead Zone/1
  PID Controller/1 -> YMC.YawMoment/1, MATLAB Function/1(YMC), Yaw_moment/1  "YM"
  vx [m/s]/1 -> Reference YR generaator/1(vx)
  Reference YR generaator/1(yr_ref) -> YMC.YaweRateReference/1, Sum/1
  Sum/1 -> YMC.YawRateError/1, PID Controller/1  "yr_e"
  "gainPI "/1 -> Demux/1
  Demux/1 -> toRTDBc1/1, PID Controller/2
  Demux/2 -> toRTDBc/1, PID Controller/3
  Steering demands [rad]/1 -> WA_estimation/1(steering_request [rad/s]), [steering]
  Yaw Rate [rad/s]/1 -> Sum/2
  Dead Zone/1 -> Demux4/1, deltaTorque [Nm]/1
  Demux4/2 -> toRTDBc23/1
  Demux4/1 -> toRTDBc22/1
  Demux4/3 -> toRTDBc20/1
  Demux4/4 -> toRTDBc21/1
  WA_estimation/1(delta [rad/s]) -> Reference YR generaator/2(delta), MATLAB Function/2(delta)

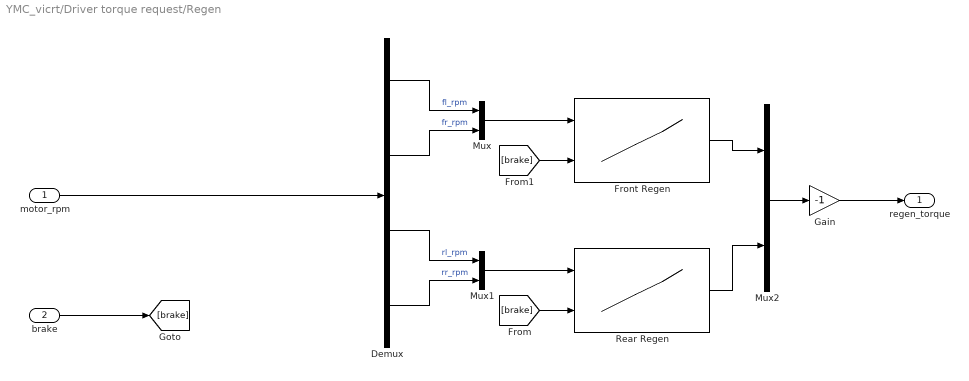
== system YMC_vicrt/Driver torque request/Regen ==
  motor_rpm : Inport
  brake : Inport  Port=2
  Demux : Demux
  Front Regen : Lookup_n-D  BreakpointsForDimension1=speedVector  BreakpointsForDimension2=brakeVector  Table=TorqueFrontRegen  InternalRulePriority=Speed  RndMeth=Simplest  InputSameDT=on
      settings: InputPortMap=u0,u1
  Gain : Gain  Gain=-1
  Mux : Mux  Inputs=2
  Mux1 : Mux  Inputs=2
  Mux2 : Mux  Inputs=2
  "Rear Regen " : Lookup_n-D  BreakpointsForDimension1=speedVector  BreakpointsForDimension2=brakeVector  Table=TorqueRearRegen  InternalRulePriority=Speed  RndMeth=Simplest  InputSameDT=on
      settings: InputPortMap=u0,u1
  regen_torque : Outport
  wires:
  motor_rpm/1 -> Demux/1
  Demux/4 -> Mux1/2  "rr_rpm"
  Demux/2 -> Mux/2  "fr_rpm"
  Mux/1 -> Front Regen/1
  Demux/1 -> Mux/1  "fl_rpm"
  Demux/3 -> Mux1/1  "rl_rpm"
  Mux1/1 -> "Rear Regen "/1
  Mux2/1 -> Gain/1
  "Rear Regen "/1 -> Mux2/2
  Front Regen/1 -> Mux2/1
  brake/1 -> [brake]
  [brake] -> "Rear Regen "/2
  [brake] -> Front Regen/2
  Gain/1 -> regen_torque/1

== system YMC_vicrt/Driver torque request/Torque Limit ==
  motor_rpm : Inport
  1-D Lookup Table : Lookup_n-D  NumberOfTableDimensions=1  BreakpointsForDimension1=speedVector  Table=TorqueLimit  InternalRulePriority=Speed  RndMeth=Simplest  InputSameDT=on
  limit_torque : Outport
  wires:
  1-D Lookup Table/1 -> limit_torque/1
  motor_rpm/1 -> 1-D Lookup Table/1

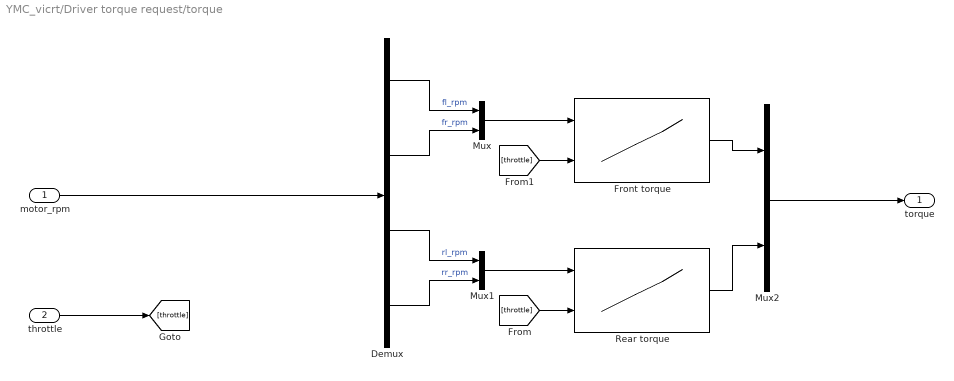
== system YMC_vicrt/Driver torque request/torque ==
  motor_rpm : Inport
  throttle : Inport  Port=2
  Demux : Demux
  Front torque : Lookup_n-D  BreakpointsForDimension1=speedVector  BreakpointsForDimension2=brakeVector  Table=TorqueFront  InternalRulePriority=Speed  RndMeth=Simplest  InputSameDT=on
      settings: InputPortMap=u0,u1
  Mux : Mux  Inputs=2
  Mux1 : Mux  Inputs=2
  Mux2 : Mux  Inputs=2
  Rear torque : Lookup_n-D  BreakpointsForDimension1=speedVector  BreakpointsForDimension2=brakeVector  Table=TorqueRear  InternalRulePriority=Speed  RndMeth=Simplest  InputSameDT=on
      settings: InputPortMap=u0,u1
  torque : Outport
  wires:
  motor_rpm/1 -> Demux/1
  Demux/4 -> Mux1/2  "rr_rpm"
  Demux/2 -> Mux/2  "fr_rpm"
  Mux/1 -> Front torque/1
  Demux/1 -> Mux/1  "fl_rpm"
  Demux/3 -> Mux1/1  "rl_rpm"
  Mux1/1 -> Rear torque/1
  Rear torque/1 -> Mux2/2
  Front torque/1 -> Mux2/1
  throttle/1 -> [throttle]
  [throttle] -> Rear torque/2
  [throttle] -> Front torque/2
  Mux2/1 -> torque/1

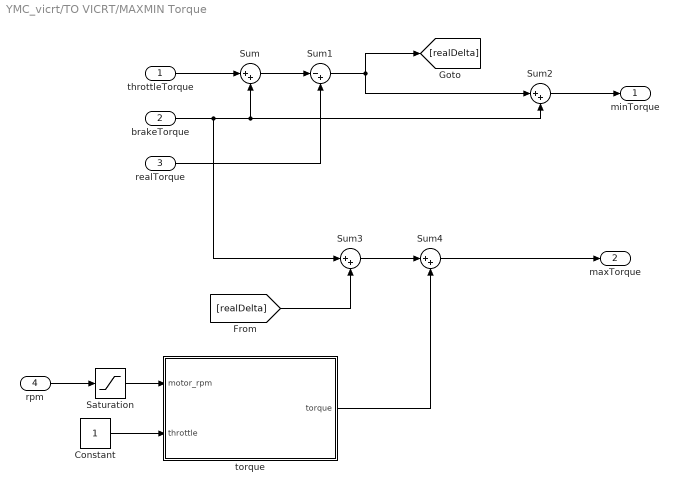
== system YMC_vicrt/TO VICRT/MAXMIN Torque ==
  throttleTorque : Inport
  brakeTorque : Inport  Port=2
  realTorque : Inport  Port=3
  rpm : Inport  Port=4
  Constant : Constant
  Saturation : Saturate  UpperLimit=20000  LowerLimit=0
  Sum{,2..4} (4 alike) : Sum  Inputs=|++
  Sum1 : Sum  Inputs=|-+
  torque : Subsystem
  minTorque : Outport
  maxTorque : Outport  Port=2
  wires:
  throttleTorque/1 -> Sum/1
  brakeTorque/1 -> Sum3/1, Sum2/2, Sum/2
  Sum/1 -> Sum1/1
  realTorque/1 -> Sum1/2
  Sum1/1 -> Sum2/1, [realDelta]
  Sum2/1 -> minTorque/1
  Sum4/1 -> maxTorque/1
  [realDelta] -> Sum3/2
  torque/1(torque) -> Sum4/2
  rpm/1 -> Saturation/1
  Saturation/1 -> torque/1(motor_rpm)
  Constant/1 -> torque/2(throttle)
  Sum3/1 -> Sum4/1

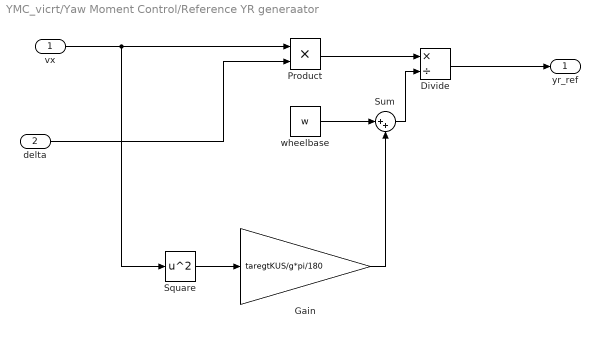
== system YMC_vicrt/Yaw Moment Control/Reference YR generaator ==
  vx : Inport
  delta : Inport  Port=2
  Divide : Product  Inputs=*/
  Gain : Gain  Gain=taregtKUS/g*pi/180
  Product : Product
  Square : Math  Operator=square  SaturateOnIntegerOverflow=on
  Sum : Sum  Inputs=|++
  wheelbase : Constant  Value=w
  yr_ref : Outport
  wires:
  vx/1 -> Square/1, Product/1
  Product/1 -> Divide/1
  Divide/1 -> yr_ref/1
  wheelbase/1 -> Sum/1
  delta/1 -> Product/2
  Square/1 -> Gain/1
  Gain/1 -> Sum/2
  Sum/1 -> Divide/2

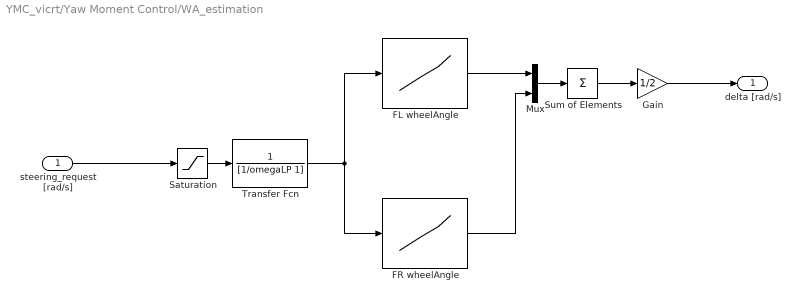
== system YMC_vicrt/Yaw Moment Control/WA_estimation ==
  steering_request [rad/s] : Inport
  FL wheelAngle : Lookup_n-D  NumberOfTableDimensions=1  BreakpointsForDimension1=steerFront(:,1)*(pi/180)  Table=steerFront(:,2)*(pi/180)  InternalRulePriority=Speed  RndMeth=Simplest  InputSameDT=on
  FR wheelAngle : Lookup_n-D  NumberOfTableDimensions=1  BreakpointsForDimension1=steerFront(:,1)*(pi/180)  Table=steerFront(:,3)*(pi/180)  InternalRulePriority=Speed  RndMeth=Simplest  InputSameDT=on
  Gain : Gain  Gain=1/2
  Mux : Mux  Inputs=2
  Saturation : Saturate  UpperLimit=95*pi/180  LowerLimit=-95*pi/180
  Sum of Elements : Sum  Inputs=+
  Transfer Fcn : TransferFcn  Denominator=[1/omegaLP 1]
  delta [rad/s] : Outport
  wires:
  FR wheelAngle/1 -> Mux/2
  Transfer Fcn/1 -> FL wheelAngle/1, FR wheelAngle/1
  Sum of Elements/1 -> Gain/1
  Gain/1 -> delta [rad/s]/1
  Mux/1 -> Sum of Elements/1
  FL wheelAngle/1 -> Mux/1
  Saturation/1 -> Transfer Fcn/1
  steering_request [rad/s]/1 -> Saturation/1

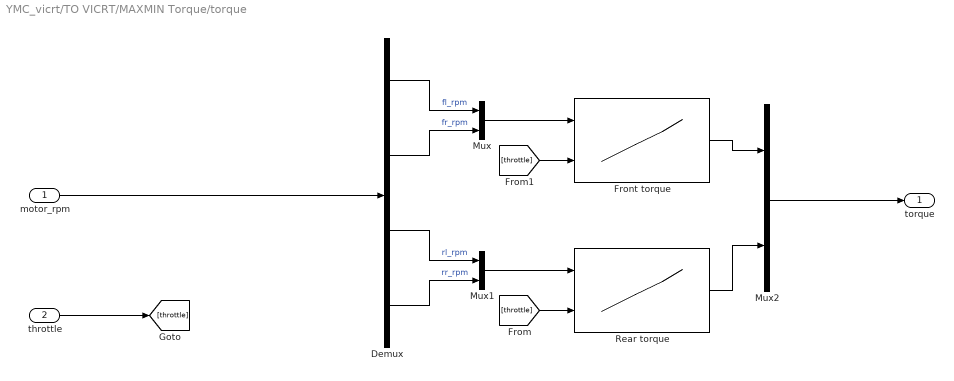
== system YMC_vicrt/TO VICRT/MAXMIN Torque/torque ==
  motor_rpm : Inport
  throttle : Inport  Port=2
  Demux : Demux
  Front torque : Lookup_n-D  BreakpointsForDimension1=speedVector  BreakpointsForDimension2=brakeVector  Table=TorqueFront  InternalRulePriority=Speed  RndMeth=Simplest  InputSameDT=on
      settings: InputPortMap=u0,u1
  Mux : Mux  Inputs=2
  Mux1 : Mux  Inputs=2
  Mux2 : Mux  Inputs=2
  Rear torque : Lookup_n-D  BreakpointsForDimension1=speedVector  BreakpointsForDimension2=brakeVector  Table=TorqueRear  InternalRulePriority=Speed  RndMeth=Simplest  InputSameDT=on
      settings: InputPortMap=u0,u1
  torque : Outport
  wires:
  motor_rpm/1 -> Demux/1
  Demux/4 -> Mux1/2  "rr_rpm"
  Demux/2 -> Mux/2  "fr_rpm"
  Mux/1 -> Front torque/1
  Demux/1 -> Mux/1  "fl_rpm"
  Demux/3 -> Mux1/1  "rl_rpm"
  Mux1/1 -> Rear torque/1
  Rear torque/1 -> Mux2/2
  Front torque/1 -> Mux2/1
  throttle/1 -> [throttle]
  [throttle] -> Rear torque/2
  [throttle] -> Front torque/2
  Mux2/1 -> torque/1

== matlab function YMC_vicrt/MATLAB Function ==
  data: kp output; vx input; ki output; BP parameter; phaseMargin parameter; m parameter; Izz parameter; a parameter; b parameter; w parameter; Cf parameter; Cr parameter
function [kp,ki] = PIsynthesis(vx, BP, phaseMargin, m, Izz, a, b, w, Cf, Cr)
% function [kp,ki] = PIsyntesis(vx, wgc, phim, m, Izz, a, b, w, Cf, Cr, Ts)
%PIDESIGN Summary of this function goes here
%   'wgc' : desired bandwidth in rad/s
%   'phim' : phase margin in rad
%   'gainPlant' : static gain of the plant(impianto) transfer function
%   'tausPlant' : poles of the plant transfer function
%   'timeC' : discrete control time

B = (Izz * (Cf + Cr) + m*(Cf*a^2+Cr*b^2)) / (m*Izz*vx);
C = (m*vx^2 *(b*Cr-a*Cf) + Cf*Cr*w^2 ) / (m*Izz*vx^2);

%% Transfer function

 s = BP*1i; % variabile di Laplace


% tausPlant = [roots([1/Izz (Cf + Cr)/(m*vx*Izz)]) ; roots([1 B C])];

% gainPlant = - tausPlant(1)/(tausPlant(2)*tausPlant(3))/Izz;

%%%
% Plant transfer function
Plant    = (s/Izz + (Cf + Cr)/(m*vx*Izz))*...
                (1/(s^2 + B*s + C));

%%%
% Get delta_K and delta_phi
magP = abs(Plant);
phaP = angle(Plant);   

deltaK      = 1/magP;
deltaPhi    = max(-pi/2, -pi + phaseMargin - phaP);


%%%
% Get kp e ki of the PI
kp          = deltaK*cos(deltaPhi);
ki          = -BP*deltaK*sin(deltaPhi);

end

== matlab function YMC_vicrt/Torque limitation/MATLAB Function ==
  data: motorTorque input; YMCtorque output; motorTorqueLimit input; YM input
function YMCtorque = torqueOptimiaztion(motorTorque, motorTorqueLimit, YM)

YMCtorque = motorTorque;

if YM > 0 
    % Adattamento coppie FRONT
    if motorTorque(2) > motorTorqueLimit(2) % Controllo FR
        YMCtorque(2) = motorTorqueLimit(2);
        YMCtorque(1) = motorTorque(1) - (motorTorque(2) - motorTorqueLimit(2));
        YMCtorque(1) = max(-motorTorqueLimit(1), YMCtorque(1));
    end

    if motorTorque(1) < -motorTorqueLimit(1) % Controllo FL
        YMCtorque(1) = -motorTorqueLimit(1);
        YMCtorque(2) = motorTorque(2) - (motorTorque(1) - motorTorqueLimit(1));
        YMCtorque(2) = min(motorTorqueLimit(2), YMCtorque(2));
    end

    % Adattamento coppie REAR
    if motorTorque(4) > motorTorqueLimit(4) % Controllo RR
        YMCtorque(4) = motorTorqueLimit(4);
        YMCtorque(3) = motorTorque(3) - (motorTorque(4) - motorTorqueLimit(4));
        YMCtorque(3) = max(-motorTorqueLimit(3), YMCtorque(3));
    end

    if motorTorque(3) < -motorTorqueLimit(3) % Controllo RL
        YMCtorque(3) = -motorTorqueLimit(3);
        YMCtorque(4) = motorTorque(4) - (motorTorque(3) - motorTorqueLimit(3));
        YMCtorque(4) = min(motorTorqueLimit(4), YMCtorque(4));
    end
end


if YM < 0

    % Adattamento coppie FRONT
     if motorTorque(1) > motorTorqueLimit(1) % Controllo FL
        YMCtorque(1) = motorTorqueLimit(1);
        YMCtorque(2) = motorTorque(2) - (motorTorque(1) - motorTorqueLimit(1));
        YMCtorque(2) = max(-motorTorqueLimit(2), YMCtorque(2));
     end

    if motorTorque(2) < -motorTorqueLimit(2) % Controllo FR
        YMCtorque(2) = -motorTorqueLimit(2);
        YMCtorque(1) = motorTorque(1) - (motorTorque(2) + motorTorqueLimit(2));
        YMCtorque(1) = min(motorTorqueLimit(1), YMCtorque(1));
    end

    % Adattamento coppie REAR
    if motorTorque(3) > motorTorqueLimit(3) % Controllo RL
        YMCtorque(3) = motorTorqueLimit(3);
        YMCtorque(4) = motorTorque(4) - (motorTorque(3) - motorTorqueLimit(3));
        YMCtorque(4) = max(-motorTorqueLimit(4), YMCtorque(4));
    end

    if motorTorque(4) < -motorTorqueLimit(4) % Controllo RR
        YMCtorque(4) = -motorTorqueLimit(4);
        YMCtorque(3) = motorTorque(3) - (motorTorque(4) - motorTorqueLimit(4));
        YMCtorque(3) = min(motorTorqueLimit(3), YMCtorque(3));
    end
  
    
end

== matlab function YMC_vicrt/Yaw Moment Control/MATLAB Function ==
  data: YMC input; YMCTorque output; tFront parameter; tRear parameter; nominalWheelRadius parameter; tau parameter; delta input
function YMCTorque = deltaMotorTorque(YMC, tFront, tRear, nominalWheelRadius, tau, delta)

csi = 0.2;

YMCFront = csi * YMC;

frontWheelForce = YMCFront / (tFront/2) / cos(delta);

frontMotorTorque = frontWheelForce * nominalWheelRadius / tau;

YMCRear = (1-csi) * YMC;

rearWheelForce = YMCRear / (tRear/2);

rearMotorTorque = rearWheelForce * nominalWheelRadius / tau;

YMCTorque = [-frontMotorTorque/2 frontMotorTorque/2 -rearMotorTorque/2 rearMotorTorque/2]';
